simulink model "Walsh06_Class_2017"  (R2017a)
settings: Solver=VariableStepAuto  StartTime=0.0  StopTime=96  RelTol=1e-3
settings Model: Creator=alexandr.lanin  LastModifiedBy=alexandr.lanin

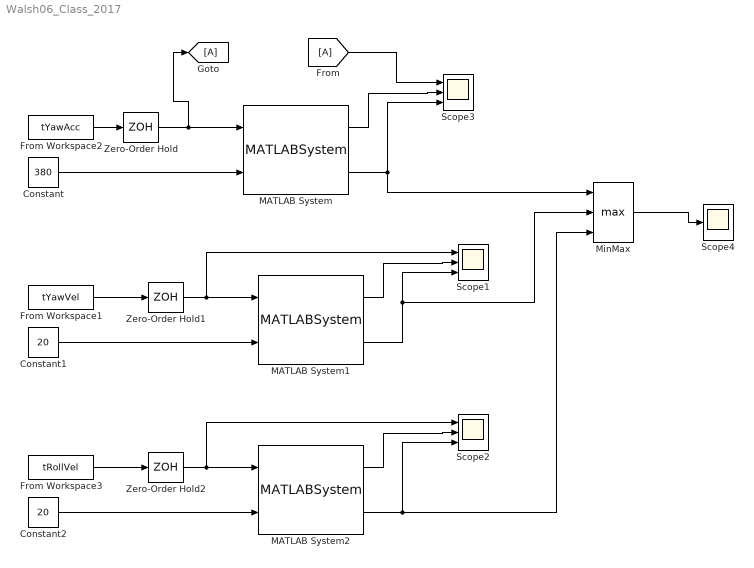
== system Walsh06_Class_2017 ==
  Constant : Constant  Value=380
  Constant1 : Constant  Value=20
  Constant2 : Constant  Value=20
  From Workspace1 : FromWorkspace  VariableName=tYawVel  SampleTime=0
  From Workspace2 : FromWorkspace  VariableName=tYawAcc  SampleTime=0
  From Workspace3 : FromWorkspace  VariableName=tRollVel  SampleTime=0
  MATLAB System : MATLABSystem  System=WolchSimCode  kMul=100  SimulateUsing=Code generation
      mask Type: WolchSimCode
      mask Display:
      | disp('WolchSimCode');
      | port_label('input',1,'u');
      | port_label('input',2,'norm');
      | port_label('output',1,'Y');
      | port_label('output',2,'Ynorm');
  MATLAB System1 : MATLABSystem  System=WolchSimCode  kMul=100  SimulateUsing=Code generation
      mask Type: WolchSimCode
      mask Display:
      | disp('WolchSimCode');
      | port_label('input',1,'u');
      | port_label('input',2,'norm');
      | port_label('output',1,'Y');
      | port_label('output',2,'Ynorm');
  MATLAB System2 : MATLABSystem  System=WolchSimCode  kMul=100  SimulateUsing=Code generation
      mask Type: WolchSimCode
      mask Display:
      | disp('WolchSimCode');
      | port_label('input',1,'u');
      | port_label('input',2,'norm');
      | port_label('output',1,'Y');
      | port_label('output',2,'Ynorm');
  MinMax : MinMax  Function=max  Inputs=3
  Scope1 : Scope  NumInputPorts=3
  Scope2 : Scope  NumInputPorts=3
  Scope3 : Scope  NumInputPorts=3
  Scope4 : Scope
  Zero-Order Hold : ZeroOrderHold  SampleTime=0.01
  Zero-Order Hold1 : ZeroOrderHold  SampleTime=0.01
  Zero-Order Hold2 : ZeroOrderHold  SampleTime=0.01
  wires:
  From Workspace2/1 -> Zero-Order Hold/1
  Zero-Order Hold/1 -> [A], MATLAB System/1
  MATLAB System/1 -> Scope3/2
  MATLAB System/2 -> MinMax/1, Scope3/3
  Constant/1 -> MATLAB System/2
  MATLAB System1/2 -> Scope1/3, MinMax/2
  Constant1/1 -> MATLAB System1/2
  MATLAB System1/1 -> Scope1/2
  From Workspace1/1 -> Zero-Order Hold1/1
  Zero-Order Hold1/1 -> Scope1/1, MATLAB System1/1
  MATLAB System2/1 -> Scope2/2
  From Workspace3/1 -> Zero-Order Hold2/1
  MATLAB System2/2 -> MinMax/3, Scope2/3
  Zero-Order Hold2/1 -> Scope2/1, MATLAB System2/1
  Constant2/1 -> MATLAB System2/2
  [A] -> Scope3/1
  MinMax/1 -> Scope4/1
